simulink model "Lab2_Counter"  (R2024a)
settings: Solver=VariableStepAuto  StartTime=0.0  StopTime=inf  RelTol=1e-3
settings Model: Creator=VICTUS  LastModifiedBy=VICTUS

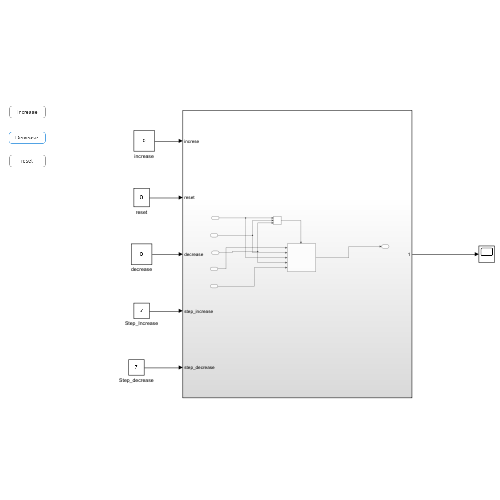
[thumbnail: Simulink's stored preview of the top-level diagram]
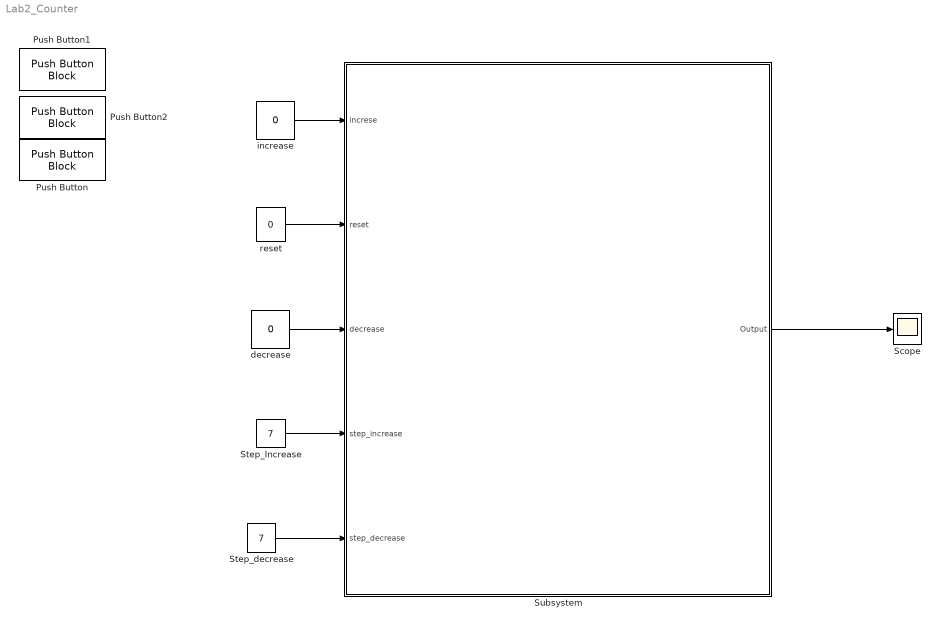
== system Lab2_Counter ==
  Push Button : PushButtonBlock  ButtonText=reset  OffValue=0.000000
  Push Button1 : PushButtonBlock  ButtonText=Increase  OffValue=0.000000
  Push Button2 : PushButtonBlock  ButtonText=Decrease  OffValue=0.000000
  Scope : Scope
  Step_Increase : Constant  Value=7
  Step_decrease : Constant  Value=7
  Subsystem : Subsystem
  decrease : Constant  Value=0  VectorParams1D=off  SampleTime=-1
  increase : Constant  Value=0  VectorParams1D=off  SampleTime=-1
  reset : Constant  Value=0
  wires:
  increase/1 -> Subsystem/1(increse)
  reset/1 -> Subsystem/2(reset)
  decrease/1 -> Subsystem/3(decrease)
  Step_Increase/1 -> Subsystem/4(step_increase)
  Step_decrease/1 -> Subsystem/5(step_decrease)
  Subsystem/1(Output) -> Scope/1

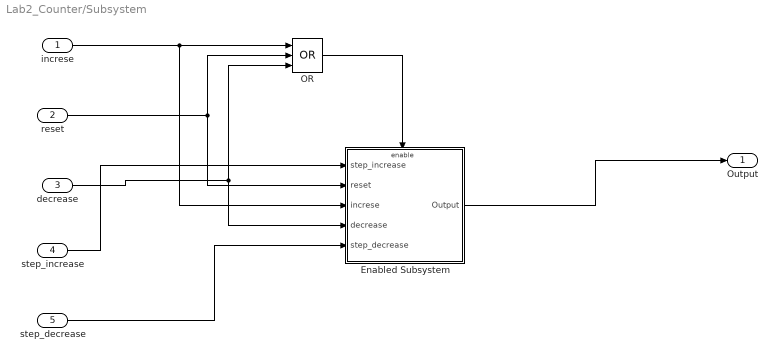
== system Lab2_Counter/Subsystem ==
  increse : Inport
  reset : Inport  Port=2
  decrease : Inport  Port=3
  step_increase : Inport  Port=4
  step_decrease : Inport  Port=5
  Enabled Subsystem : Subsystem  TreatAsAtomicUnit=on
  OR : Logic  Operator=OR  Inputs=3  AllPortsSameDT=off  OutDataTypeStr=boolean
  Output : Outport
  wires:
  decrease/1 -> Enabled Subsystem/4(decrease), OR/3
  step_decrease/1 -> Enabled Subsystem/5(step_decrease)
  reset/1 -> OR/2, Enabled Subsystem/2(reset)
  Enabled Subsystem/1(Output) -> Output/1
  increse/1 -> Enabled Subsystem/3(increse), OR/1
  OR/1 -> Enabled Subsystem/Enable
  step_increase/1 -> Enabled Subsystem/1(step_increase)

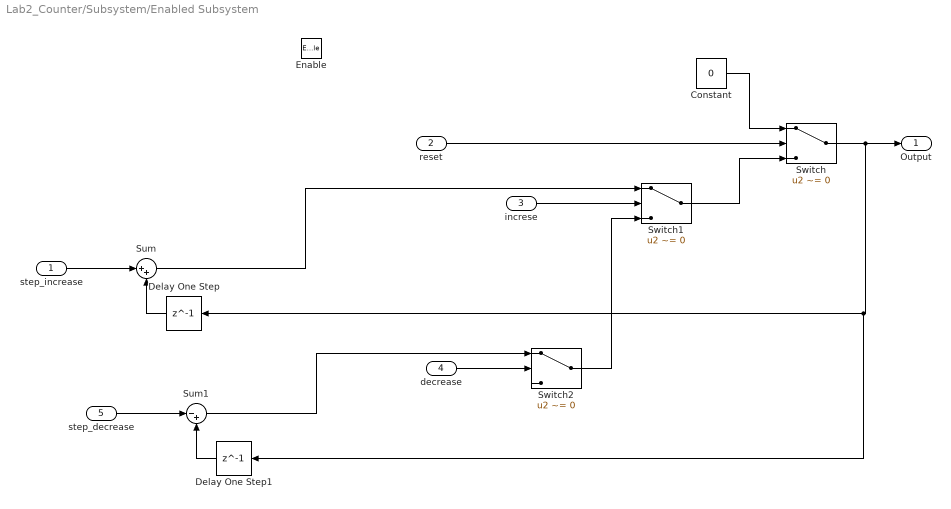
== system Lab2_Counter/Subsystem/Enabled Subsystem ==
  step_increase : Inport
  reset : Inport  Port=2
  increse : Inport  Port=3
  decrease : Inport  Port=4
  step_decrease : Inport  Port=5
  Enable : EnablePort
  Constant : Constant  Value=0
  Delay One Step : Delay  DelayLength=1
  Delay One Step1 : Delay  DelayLength=1
  Sum : Sum  Inputs=|++
  Sum1 : Sum  Inputs=|-+
  Switch : Switch  Criteria=u2 ~= 0  SaturateOnIntegerOverflow=off  InputSameDT=off
  Switch1 : Switch  Criteria=u2 ~= 0  SaturateOnIntegerOverflow=off  InputSameDT=off
  Switch2 : Switch  Criteria=u2 ~= 0  SaturateOnIntegerOverflow=off  InputSameDT=off
  Output : Outport
  wires:
  Delay One Step/1 -> Sum/2
  step_increase/1 -> Sum/1
  reset/1 -> Switch/2
  Switch/1 -> Delay One Step1/1, Delay One Step/1, Output/1
  Constant/1 -> Switch/1
  step_decrease/1 -> Sum1/1
  Delay One Step1/1 -> Sum1/2
  increse/1 -> Switch1/2
  Sum/1 -> Switch1/1
  Switch1/1 -> Switch/3
  decrease/1 -> Switch2/2
  Switch2/1 -> Switch1/3
  Sum1/1 -> Switch2/1
